simulink model "usrp_fm_fdm"  (R2014b)
settings: Solver=ode45  StartTime=0.0  StopTime=inf  RelTol=1e-3
PreLoadFcn:
  | %%%%%%%%%%%%%%%%%%%%%%%%%%%%%%%%%%%%%%%%%%%%%%%%%%%%%%%%%%%%%%%%%%%%%%%%%%%
  | % check to see if Simulink library folder is missing from the MATLAB path %
  | %%%%%%%%%%%%%%%%%%%%%%%%%%%%%%%%%%%%%%%%%%%%%%%%%%%%%%%%%%%%%%%%%%%%%%%%%%%
  | if isempty(strfind(path, 'rtlsdr_book_library'))
  | 
  |     % create error window
  |     fig_error = figure(...
  |         'Name', 'Error: RTL-SDR Book Library',...
  |         'Toolbar','none',...
  |         'MenuBar','none',...
  |         'NumberTitle','off',...
  |         'Resize','off',...
  |         'WindowStyle','modal');
  |     fig_error.Position(3) = 600;
  |     fig_error.Position(4) = 150;
  |     fig_axes = axes(...
  |         'Parent',fig_error,...
  |         'Position',[0,0,1,1],...
  |         'visible','off');
  |     % error message
  |     t_title = text(.05,.8,...
  |         'MISSING DIRECTORIES',...
  |         'FontSize',11.5);
  |     t_body = text(.075,.6,...
  |         [{'Simulink cannot find the  \it{<root>}\rm / \it{rtlsdr\_book\_library}\rm  folder in the \it{MATLAB Path}\rm.'},...
  |         {'Please set the MATLAB path following the instructions given in Exercise 2.4.'}],...
  |         'FontSize',10.5);
  |     % buttons
  |     btn_path = uicontrol(...
  |         'Parent',fig_error,...
  |         'String','Set Path Now',...
  |         'FontSize',10,...
  |         'Callback', 'pathtool; close(fig_error);',...
  |         'Position', [fig_error.Position(3)/2-210, 30, 200, 30]);
  |     btn_abort = uicontrol(...
  |         'Parent',fig_error,...
  |         'String','No thanks',...
  |         'FontSize',10,...
  |         'Callback', 'close(fig_error); abort=1;',...
  |         'Position', [fig_error.Position(3)/2+10, 30, 200, 30]);
  | 
  |     % pause to allow user to interact with error box
  |     uiwait(fig_error);
  | 
  |     % abort simulation
  |     try
  |         if abort==1
  |             set_param(gcs, 'SimulationCommand', 'stop');
  |         end
  |     end
  | 
  |     % if user has set path, allow diagram to be updated
  |     if ~exist('abort','var')
  |         % create error window
  |         fig_update = figure(...
  |             'Name', 'Update Diagram',...
  |             'Toolbar','none',...
  |             'MenuBar','none',...
  |             'NumberTitle','off',...
  |             'Resize','off');
  |         fig_update.Position(3) = 400;
  |         fig_update.Position(4) = 120;
  |         fig_axes = axes(...
  |             'Parent',fig_update,...
  |             'Position',[0,0,1,1],...
  |             'visible','off');
  |         % instruction message
  |         t_body = text(.075,.7,...
  |             'Once you have set the path, update the block diagram',...
  |             'FontSize',10.5);
  |         % button
  |         btn_update = uicontrol(...
  |             'Parent',fig_update,...
  |             'String','Update Block Diagram',...
  |             'FontSize',10,...
  |             'Callback', 'set_param(gcs,''SimulationCommand'',''update''); close(gcf)',...
  |             'Position', [fig_update.Position(3)/2-100, 30, 200, 30]);
  |     end
  | 
  |     % clear error components
  |     clear('fig_error','fig_update','fig_axes','t_title','t_body','btn_path','btn_abort','btn_update','abort');
  | 
  | end
  | %%%%%%%%%%%%%%%%%%%%%%%%%%%%%%%%%%%%%%%%%%%%%%%%%%%%%%%%%%%%%%%%%%%%%%%%%%%
undefined symbols (not defined in the file): dfilt, fdesignblkfcn, gcbh, startfcn_spectrum_analyzer
libraries: dsparch4 x9, dspmlti4 x4, dspvision x4, dspsrcs4 x4, dspmtrx3 x2, rtlsdr_book_library x1, commsdrhw_v2 x1
(part 1 of 2)
CloseFcn:
  | closefcn_model
Description:
  | Software, Simulation Examples and Design Exercises Licence Agreement
  | 
  | This license agreement refers to the simulation examples, design exercises and files,
  | and associated software MATLAB and Simulink resources that accompany the book:
  | 
  |      Title: Software Defined Radio using MATLAB & Simulink and the RTL-SDR
  |      Published by Strathclyde Academic Media, 2015
  |      Authored by Robert W. Stewart, Kenneth W. Barlee, Dale S.W. Atkinson,
  |      and Louise H. Crockett
  | 
  | and made available as a download from, www.desktopSDR.com or variously acquired
  | by other means such as via USB storage, cloud storage, disk or any other electronic
  | or optical or magnetic storage mechanism. These files and associated software may
  | be used subject to the terms of agreement of the conditions below:
  | 
  |     Copyright © 2015 Robert W. Stewart, Kenneth W. Barlee, Dale S.W. Atkinson,
  |     and Louise H. Crockett
  |     All rights reserved.
  | 
  | Redistribution and use in source and binary forms, with or without modification, are
  | permitted provided that the following conditions are met:
  | 
  |    1.  Redistributions of source code must retain the above copyright notice, this list of
  |         conditions and the following disclaimer.
  | 
  |    2.  Redistributions in binary form must reproduce the above copyright notice, this
  |         list of conditions and the following disclaimer in the documentation and/or other
  |         materials provided with the distribution.
  | 
  |    3.  Neither the name of the copyright holder nor the names of its contributors may
  |         be used to endorse or promote products derived from this software without
  |         specific prior written permission.
  | 
  |    4.  In all cases, the software is, and all modifications and derivatives of the
  |         software shall be, licensed to you solely for use in conjunction with The
  |         MathWorks, Inc. products and service offerings.
  | 
  | THIS SOFTWARE IS PROVIDED BY THE COPYRIGHT HOLDERS AND CONTRIBUTORS
  | "AS IS" AND ANY EXPRESS OR IMPLIED WARRANTIES, INCLUDING, BUT NOT LIMITED
  | TO, THE IMPLIED WARRANTIES OF MERCHANTABILITY AND FITNESS FOR A
  | PARTICULAR PURPOSE ARE DISCLAIMED. IN NO EVENT SHALL THE COPYRIGHT
  | HOLDER OR CONTRIBUTORS BE LIABLE FOR ANY DIRECT, INDIRECT, INCIDENTAL,
  | SPECIAL, EXEMPLARY, OR CONSEQUENTIAL DAMAGES (INCLUDING, BUT NOT
  | LIMITED TO, PROCUREMENT OF SUBSTITUTE GOODS OR SERVICES; LOSS OF USE,
  | DATA, OR PROFITS; OR BUSINESS INTERRUPTION) HOWEVER CAUSED AND ON ANY
  | THEORY OF LIABILITY, WHETHER IN CONTRACT, STRICT LIABILITY, OR TORT
  | (INCLUDING NEGLIGENCE OR OTHERWISE) ARISING IN ANY WAY OUT OF THE USE
  | OF THIS SOFTWARE, EVEN IF ADVISED OF THE POSSIBILITY OF SUCH DAMAGE.
  | 
  | 
  | Audio Tracks used in Simulations Examples and Design Exercises
  | 
  | The music and vocal files used within the Examples files and software within the book
  | were variously written, arranged, performed, recorded and produced by Garrey Rice,
  | Adam Struth, Jamie Struth, Iain Thistlethwaite and also Marshall Craigmyle who
  | collectively, and individually where appropriate, assert and retain all of their copyright,
  | performance and artistic rights. Permission to use and reproduce this music is
  | granted for all purposes associated with MATLAB and Simulink software and the
  | simulation examples and design exercises files that accompany this book. Requests to
  | use the music for any other purpose should be directed to: info@desktopSDR.com.
  | For information on music track names, full credits, and links to the musicians please
  | refer to www.desktopSDR.com/more/audio.
settings Model: SimulationMode=accelerator  Creator=desktopSDR Team  LastModifiedBy=desktopSDR Team
settings DataIOCC: LimitDataPoints=off  SaveOutput=off  SignalLogging=off  SaveTime=off

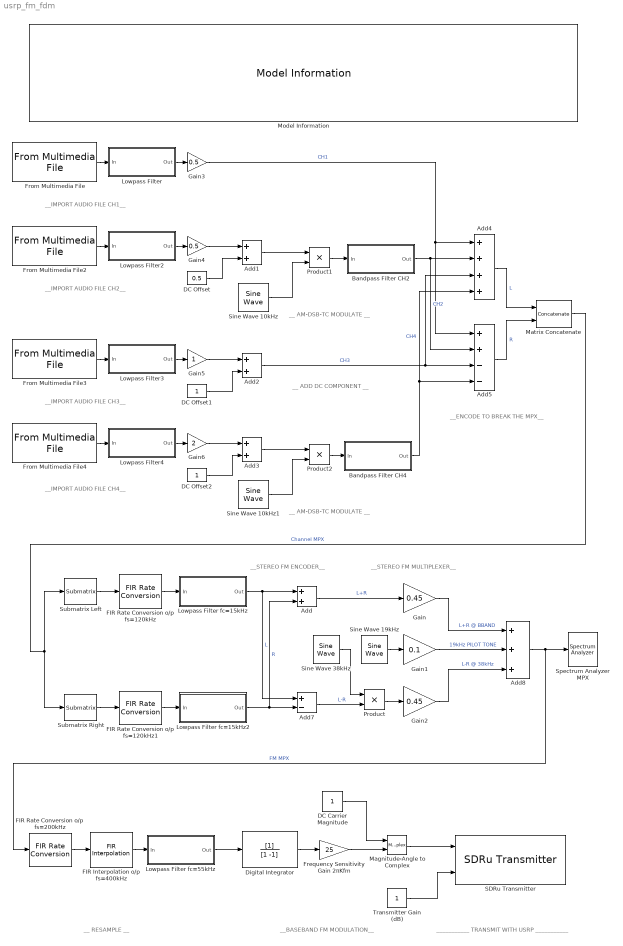
== system usrp_fm_fdm ==
  note: __ AM-DSB-TC MODULATE __
  note: __ AM-DSB-TC MODULATE __
  note: __ ADD DC COMPONENT __
  note: __IMPORT AUDIO FILE CH1__
  note: __IMPORT AUDIO FILE CH2__
  note: __IMPORT AUDIO FILE CH3__
  note: __IMPORT AUDIO FILE CH4__
  note: __ENCODE TO BREAK THE MPX__
  note: __STEREO FM MULTIPLEXER__
  note: __STEREO FM ENCODER__
  note: __ RESAMPLE __
  note: ___________ TRANSMIT WITH USRP ___________
  note: __BASEBAND FM MODULATION__
  Add{,1..3} (4 alike) : Sum
  Add4 : Sum  Inputs=++++
  Add5 : Sum  Inputs=++--
  Add7 : Sum  Inputs=+-
  Add8 : Sum  Inputs=+++
  Bandpass Filter CH2 : Subsystem  DialogController=fdesignblkfcn  InitFcn=fdesignblkfcn(gcbh, {'InitFcn'});  mask(Bandpass Filter){}
      mask help: Design a bandpass filter
      settings: CopyFcn=fdesignblkfcn(gcbh, {'CopyFcn'});
      mask Help: helpview(mapfilelocation('dsp'), 'dspbandpassfilter');
      mask Display: disp('Bandpass');
  Bandpass Filter CH4 : Subsystem  DialogController=fdesignblkfcn  InitFcn=fdesignblkfcn(gcbh, {'InitFcn'});  mask(Bandpass Filter){}
      mask help: Design a bandpass filter
      settings: CopyFcn=fdesignblkfcn(gcbh, {'CopyFcn'});
      mask Help: helpview(mapfilelocation('dsp'), 'dspbandpassfilter');
      mask Display: disp('Bandpass');
  DC Carrier Magnitude : Constant
  DC Offset : Constant  Value=0.5
  DC Offset1 : Constant
  DC Offset2 : Constant
  Digital Integrator : DiscreteFilter  Denominator=[1 -1]  InputProcessing=Columns as channels (frame based)  FilterStructure=Direct form II transposed  a0EqualsOne=on
  FIR Interpolation o/p fs=400kHz : dspmlti4/FIR Interpolation  h=firpm(100, [0 53e3 65e3 400e3/2]/(400e3/2), [1 1 0 0], [1 1],20)  L=2  framing=Allow multirate processing  outputBufInitCond=0  InputProcessing=Columns as channels (frame based)  firstCoeffDataTypeStr=Inherit: Same word length as input  firstCoeffLastDataTypeStr=Inherit: Same word length as input  firstCoeffMin=[]  firstCoeffMax=[]  outputDataTypeStr=Inherit: Same as accumulator  outputLastDataTypeStr=Inherit: Same as accumulator  outputMin=[]  outputMax=[]  roundingMode=Floor  overflowMode=off  FilterSource=Specify via dialog  FilterObject=Hm_firinterp
  FIR Rate Conversion o/p fs=120kHz : dspmlti4/FIR Rate Conversion  L=5  h=firpm(250, [0 15e3 20e3 240e3/2]/(240e3/2), [1 1 0 0], [1 1],20)  M=2  firstCoeffDataTypeStr=Inherit: Same word length as input  firstCoeffLastDataTypeStr=Inherit: Same word length as input  firstCoeffMin=[]  firstCoeffMax=[]  outputDataTypeStr=Inherit: Same as accumulator  outputLastDataTypeStr=Inherit: Same as accumulator  outputMin=[]  outputMax=[]  roundingMode=Floor  overflowMode=off  FilterSource=Specify via dialog  FilterObject=Hm_firsrc
  FIR Rate Conversion o/p fs=120kHz1 : dspmlti4/FIR Rate Conversion  L=5  h=firpm(250, [0 15e3 20e3 240e3/2]/(240e3/2), [1 1 0 0], [1 1],20)  M=2  firstCoeffDataTypeStr=Inherit: Same word length as input  firstCoeffLastDataTypeStr=Inherit: Same word length as input  firstCoeffMin=[]  firstCoeffMax=[]  outputDataTypeStr=Inherit: Same as accumulator  outputLastDataTypeStr=Inherit: Same as accumulator  outputMin=[]  outputMax=[]  roundingMode=Floor  overflowMode=off  FilterSource=Specify via dialog  FilterObject=Hm_firsrc
  FIR Rate Conversion o/p fs=200kHz : dspmlti4/FIR Rate Conversion  L=5  h=firpm(200, [0 53e3 65e3 600e3/2]/(600e3/2), [1 1 0 0], [1 1],20)  M=3  firstCoeffDataTypeStr=Inherit: Same word length as input  firstCoeffLastDataTypeStr=Inherit: Same word length as input  firstCoeffMin=[]  firstCoeffMax=[]  outputDataTypeStr=Inherit: Same as accumulator  outputLastDataTypeStr=Inherit: Same as accumulator  outputMin=[]  outputMax=[]  roundingMode=Floor  overflowMode=off  FilterSource=Specify via dialog  FilterObject=Hm_firsrc
  Frequency Sensitivity Gain 2πKfm : Gain  Gain=25
  From Multimedia File : dspvision/From Multimedia File  inputFilename=../../audio_sources/music1_mono48kHz.wav  loop=on  numPlays=inf  outputStreams=Audio only  videoDataType=single  audioDataType=double  inheritSampleTime=on  userDefinedSampleTime=1/30  noAudioOutput=off  isIntensityVideo=off  fourcc=RGB  colorVideoFormat=Separate color signals  outputEOF=off  dataOrg=Column-major  audioFrameSize=600  computeAudioFrameSize=off  outSamplingMode=Frame based
  From Multimedia File2 : dspvision/From Multimedia File  inputFilename=../../audio_sources/music2_mono48kHz.wav  loop=on  numPlays=inf  outputStreams=Audio only  videoDataType=single  audioDataType=double  inheritSampleTime=on  userDefinedSampleTime=1/30  noAudioOutput=off  isIntensityVideo=off  fourcc=RGB  colorVideoFormat=Separate color signals  outputEOF=off  dataOrg=Column-major  audioFrameSize=600  computeAudioFrameSize=off  outSamplingMode=Frame based
  From Multimedia File3 : dspvision/From Multimedia File  inputFilename=../../audio_sources/music3_mono48kHz.wav  loop=on  numPlays=inf  outputStreams=Audio only  videoDataType=single  audioDataType=double  inheritSampleTime=on  userDefinedSampleTime=1/30  noAudioOutput=off  isIntensityVideo=off  fourcc=RGB  colorVideoFormat=Separate color signals  outputEOF=off  dataOrg=Column-major  audioFrameSize=600  computeAudioFrameSize=off  outSamplingMode=Frame based
  From Multimedia File4 : dspvision/From Multimedia File  inputFilename=../../audio_sources/music4_mono48kHz.wav  loop=on  numPlays=inf  outputStreams=Audio only  videoDataType=single  audioDataType=double  inheritSampleTime=on  userDefinedSampleTime=1/30  noAudioOutput=off  isIntensityVideo=off  fourcc=RGB  colorVideoFormat=Separate color signals  outputEOF=off  dataOrg=Column-major  audioFrameSize=600  computeAudioFrameSize=off  outSamplingMode=Frame based
  Gain : Gain  Gain=0.45
  Gain1 : Gain  Gain=0.1
  Gain2 : Gain  Gain=0.45
  Gain3 : Gain  Gain=0.5
  Gain4 : Gain  Gain=0.5
  Gain5 : Gain
  Gain6 : Gain  Gain=2
  Lowpass Filter : Subsystem  DialogController=fdesignblkfcn  InitFcn=fdesignblkfcn(gcbh, {'InitFcn'});  mask(Lowpass Filter){}
      mask help: Design a lowpass filter
      settings: CopyFcn=fdesignblkfcn(gcbh, {'CopyFcn'});
      mask Help: helpview(mapfilelocation('dsp'), 'dsplowpassfilter');
      mask Display: disp('Lowpass')
  Lowpass Filter fc=15kHz : Subsystem  DialogController=fdesignblkfcn  InitFcn=fdesignblkfcn(gcbh, {'InitFcn'});  mask(Lowpass Filter){}
      mask help: Design a lowpass filter
      settings: CopyFcn=fdesignblkfcn(gcbh, {'CopyFcn'});
      mask Help: helpview(mapfilelocation('dsp'), 'dsplowpassfilter');
      mask Display: disp('Lowpass')
  Lowpass Filter fc=15kHz2 : Subsystem  DialogController=fdesignblkfcn  InitFcn=fdesignblkfcn(gcbh, {'InitFcn'});  mask(Lowpass Filter){}
      mask help: Design a lowpass filter
      settings: CopyFcn=fdesignblkfcn(gcbh, {'CopyFcn'});
      mask Help: helpview(mapfilelocation('dsp'), 'dsplowpassfilter');
      mask Display: disp('Lowpass')
  Lowpass Filter fc=55kHz : Subsystem  DialogController=fdesignblkfcn  InitFcn=fdesignblkfcn(gcbh, {'InitFcn'});  mask(Lowpass Filter){}
      mask help: Design a lowpass filter
      settings: CopyFcn=fdesignblkfcn(gcbh, {'CopyFcn'});
      mask Help: helpview(mapfilelocation('dsp'), 'dsplowpassfilter');
      mask Display: disp('Lowpass')
  Lowpass Filter2 : Subsystem  DialogController=fdesignblkfcn  InitFcn=fdesignblkfcn(gcbh, {'InitFcn'});  mask(Lowpass Filter){}
      mask help: Design a lowpass filter
      settings: CopyFcn=fdesignblkfcn(gcbh, {'CopyFcn'});
      mask Help: helpview(mapfilelocation('dsp'), 'dsplowpassfilter');
      mask Display: disp('Lowpass')
  Lowpass Filter3 : Subsystem  DialogController=fdesignblkfcn  InitFcn=fdesignblkfcn(gcbh, {'InitFcn'});  mask(Lowpass Filter){}
      mask help: Design a lowpass filter
      settings: CopyFcn=fdesignblkfcn(gcbh, {'CopyFcn'});
      mask Help: helpview(mapfilelocation('dsp'), 'dsplowpassfilter');
      mask Display: disp('Lowpass')
  Lowpass Filter4 : Subsystem  DialogController=fdesignblkfcn  InitFcn=fdesignblkfcn(gcbh, {'InitFcn'});  mask(Lowpass Filter){}
      mask help: Design a lowpass filter
      settings: CopyFcn=fdesignblkfcn(gcbh, {'CopyFcn'});
      mask Help: helpview(mapfilelocation('dsp'), 'dsplowpassfilter');
      mask Display: disp('Lowpass')
  Magnitude-Angle to Complex : MagnitudeAngleToComplex
  Matrix Concatenate : Concatenate  Mode=Multidimensional array  ConcatenateDimension=2
  Model Information : rtlsdr_book_library/Additional Tools/Model Information/Model Information
  Product : Product
  Product1 : Product
  Product2 : Product
  SDRu Transmitter : commsdrhw_v2/SDRu Transmitter  rxtx=tx  platform=N200/N210/USRP2  USRP2_IP='169.254.10.2'  USRP_IP_X300='192.168.10.2'  USRP_IP_X310='192.168.10.2'  USRP_serialNumB200=''  USRP_serialNumB210=''  centerFrequency=433.9e6  centerFrequencySrc=Dialog  loOffset=1.5e6  loOffsetSrc=Dialog  masterClkRateB200=32e6  masterClkRateB210=32e6  masterClkRateX300=200e6  masterClkRateX310=200e6  masterClkRateParam=100e6  gain=10  gainSrc=Input port  decimInterp=250  decimInterpSrc=Dialog  USRP2_IP_NUM=[49 54 57 46 50 53 52 46 49 48 46 50]  frameLength=362  outputDatatype=int16  overrunUnderrunPort=off  sampleTime=1  dboardInfo=|  HOST_DATA_PORT=30000  HOST_CONTROL_PORT=30001  USRP2_DATA_PORT=32769  USRP2_CONTROL_PORT=32768  bufferMode=Continuous streaming  EnableBurstMode=off  NumFramesInBurst=100  USRP_ID='169.254.10.2'
      | dbid: 0
      |           dbName: 'no db found'
      |          freqMin: 0
      |          freqMax: 0
      |          gainMin: 0
      |          gainMax: 0
      |     gainStepSize: 0
  Sine Wave 10kHz : dspsrcs4/Sine Wave  Amplitude=1  Frequency=10e3  Phase=0  SampleMode=Discrete  OutComplex=Real  CompMethod=Trigonometric fcn  TableSize=Speed  SampleTime=1/48e3  SamplesPerFrame=600  ResetState=Restart at time zero  dataType=double  wordLen=16  udDataType=sfix(16)  fracBitsMode=Best precision  numFracBits=15  OutDataTypeStr=double  LastOutDataTypeStr=double
  Sine Wave 10kHz1 : dspsrcs4/Sine Wave  Amplitude=1  Frequency=10e3  Phase=0  SampleMode=Discrete  OutComplex=Real  CompMethod=Trigonometric fcn  TableSize=Speed  SampleTime=1/48e3  SamplesPerFrame=600  ResetState=Restart at time zero  dataType=double  wordLen=16  udDataType=sfix(16)  fracBitsMode=Best precision  numFracBits=15  OutDataTypeStr=double  LastOutDataTypeStr=double
  Sine Wave 19kHz : dspsrcs4/Sine Wave  Amplitude=1  Frequency=19e3  Phase=0  SampleMode=Discrete  OutComplex=Real  CompMethod=Trigonometric fcn  TableSize=Speed  SampleTime=1/120e3  SamplesPerFrame=1500  ResetState=Restart at time zero  dataType=double  wordLen=16  udDataType=sfix(16)  fracBitsMode=Best precision  numFracBits=15  OutDataTypeStr=double  LastOutDataTypeStr=double
  Sine Wave 38kHz : dspsrcs4/Sine Wave  Amplitude=1  Frequency=38e3  Phase=0  SampleMode=Discrete  OutComplex=Real  CompMethod=Trigonometric fcn  TableSize=Speed  SampleTime=1/120e3  SamplesPerFrame=1500  ResetState=Restart at time zero  dataType=double  wordLen=16  udDataType=sfix(16)  fracBitsMode=Best precision  numFracBits=15  OutDataTypeStr=double  LastOutDataTypeStr=double
  Spectrum Analyzer MPX : SpectrumAnalyzer  StartFcn=startfcn_spectrum_analyzer;
  Submatrix Left : dspmtrx3/Submatrix  RowSpan=All rows  RowStartMode=First  RowStartIndex=1  RowEndMode=Last  RowEndIndex=1  ColSpan=One column  ColStartMode=First  ColStartIndex=1  ColEndMode=Last  ColEndIndex=1
  Submatrix Right : dspmtrx3/Submatrix  RowSpan=All rows  RowStartMode=First  RowStartIndex=1  RowEndMode=Last  RowEndIndex=1  ColSpan=One column  ColStartMode=Last  ColStartIndex=1  ColEndMode=Last  ColEndIndex=1
  Transmitter Gain (dB) : Constant
  wires:
  From Multimedia File/1 -> Lowpass Filter/1(In)
  From Multimedia File2/1 -> Lowpass Filter2/1(In)
  Gain3/1 -> Add5/1, Add4/1  "CH1"
  Matrix Concatenate/1 -> Submatrix Right/1, Submatrix Left/1  "Channel MPX"
  Bandpass Filter CH2/1(Out) -> Add5/2, Add4/2  "CH2"
  Sine Wave 10kHz/1 -> Product1/2
  Lowpass Filter2/1(Out) -> Gain4/1
  Lowpass Filter/1(Out) -> Gain3/1
  Add4/1 -> Matrix Concatenate/1  "L"
  From Multimedia File3/1 -> Lowpass Filter3/1(In)
  From Multimedia File4/1 -> Lowpass Filter4/1(In)
  Add2/1 -> Add4/3, Add5/3  "CH3"
  Bandpass Filter CH4/1(Out) -> Add4/4, Add5/4  "CH4"
  Add5/1 -> Matrix Concatenate/2  "R"
  Digital Integrator/1 -> Frequency Sensitivity Gain 2πKfm/1
  DC Carrier Magnitude/1 -> Magnitude-Angle to Complex/1
  Frequency Sensitivity Gain 2πKfm/1 -> Magnitude-Angle to Complex/2
  FIR Rate Conversion o/p fs=200kHz/1 -> FIR Interpolation o/p fs=400kHz/1
  Submatrix Left/1 -> FIR Rate Conversion o/p fs=120kHz/1
  Magnitude-Angle to Complex/1 -> SDRu Transmitter/1
  Transmitter Gain (dB)/1 -> SDRu Transmitter/2
  FIR Interpolation o/p fs=400kHz/1 -> Lowpass Filter fc=55kHz/1(In)
  FIR Rate Conversion o/p fs=120kHz/1 -> Lowpass Filter fc=15kHz/1(In)
  FIR Rate Conversion o/p fs=120kHz1/1 -> Lowpass Filter fc=15kHz2/1(In)
  Add/1 -> Gain/1  "L+R"
  Add7/1 -> Product/2  "L-R"
  Gain/1 -> Add8/1  "L+R @ BBAND"
  Lowpass Filter fc=15kHz2/1(Out) -> Add/2, Add7/2  "R"
  Lowpass Filter fc=15kHz/1(Out) -> Add/1, Add7/1  "L"
  Sine Wave 38kHz/1 -> Product/1
  Product/1 -> Gain2/1
  Sine Wave 19kHz/1 -> Gain1/1
  Gain1/1 -> Add8/2  "19kHz PILOT TONE"
  Gain2/1 -> Add8/3  "L-R @ 38kHz"
  Add8/1 -> Spectrum Analyzer MPX/1, FIR Rate Conversion o/p fs=200kHz/1  "FM MPX"
  Lowpass Filter fc=55kHz/1(Out) -> Digital Integrator/1
  Product1/1 -> Bandpass Filter CH2/1(In)
  DC Offset/1 -> Add1/2
  Gain4/1 -> Add1/1
  Add1/1 -> Product1/1
  Lowpass Filter3/1(Out) -> Gain5/1
  Sine Wave 10kHz1/1 -> Product2/2
  Lowpass Filter4/1(Out) -> Gain6/1
  Product2/1 -> Bandpass Filter CH4/1(In)
  DC Offset2/1 -> Add3/2
  Gain6/1 -> Add3/1
  Add3/1 -> Product2/1
  DC Offset1/1 -> Add2/2
  Gain5/1 -> Add2/1
  Submatrix Right/1 -> FIR Rate Conversion o/p fs=120kHz1/1

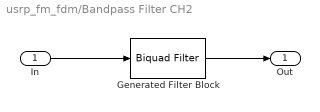
== system usrp_fm_fdm/Bandpass Filter CH2 ==
  In : Inport
  Generated Filter Block : dsparch4/Biquad Filter  Tag=BlockMethodSubSystem  IIRFiltStruct=Direct form II  CoeffSource=Specify via dialog  BiQuadCoeffs=[0.038316192503797628 0 -0.038316192503797628 1 -1.4647964271306382 0.94471193100608086;0.079066094669843018 0 -0.079066094669843018 1 -1.4478872277903871 0.92340777287438502;1.4987829140143916 0 -1.4987829140143916 1 -1.3806603018180277 0.84224281947976043;1.4262911444791151 0 -1.4262911444791151 1 0.58822635838518289 0.83492615482033594;0.12651868683152687 0 -0.12651868683152687 1 0.55132638249904864 0.75583004259253694;0.16278534730934821 0 -0.16278534730934821 1 -1.2966897472444947 0.74843901978838634;0.17165110687366142 0 -0.17165110687366142 1 -1.2286258519522211 0.67826050546120453;1.2698273089041128 0 -1.2698273089041128 1 -1.2113783161788541 0.66128071032184788;0.20679428223229873 0 -0.20679428223229873 1 0.45755483002581882 0.59529881813215735;0.24203724548995573 0 -0.24203724548995573 1 -1.1410250658492758 0.59529322698110076;0.25085765032621543 0 -0.25085765032621543 1 -1.0676878443588242 0.53197037847147466;1.126279711749548 0 -1.126279711749548 1 -1.0487453100276105 0.51650173917589026;0.28689353541085899 0 -0.28689353541085899 1 0.35194175339474887 0.46218165129526712;0.32503837865501967 0 -0.32503837865501967 1 -0.96986311471358477 0.45593385510682533;1.0469924746795094 0 -1.0469924746795094 1 -0.88468241094327671 0.39740220475460497;0.36600529716476377 0 -0.36600529716476377 1 0.28503939659387545 0.39655389906045352;0.97025355161809246 0 -0.97025355161809246 1 -0.79108046931960774 0.34121276752547225;0.41170205075459598 0 -0.41170205075459598 1 0.21209573444104943 0.33805385051512005;0.89433754435568558 0 -0.89433754435568558 1 -0.68658006847610853 0.28850567166718427;0.81944502214294834 0 -0.81944502214294834 1 0.13161626710115268 0.28686560436176478;0.46356432779720524 0 -0.46356432779720524 1 0.04162240295248873 0.24384468958098351;0.74310982737617426 0 -0.74310982737617426 1 -0.56911862362598731 0.24200449865234019;0.52401642408429905 0 -0.52401642408429905 1 -0.060257140448974872 0.21085064512665347;0.66634747068770672 0 -0.66634747068770672 1 -0.43950658142365717 0.20676604963866144;0.59171836614561379 0 -0.59171836614561379 1 -0.17601055769180649 0.19112080655833777;0.62712191993186395 0 -0.62712191993186395 1 -0.30478008617749786 0.1889115855767009;0.6996674218388591 0 -0.6996674218388591 1 -0.23904135382384295 0.18757452699095289;0.5533055925452488 0 -0.5533055925452488 1 -0.11634228576068448 0.19906897851393116;0.7691707424752533 0 -0.7691707424752533 1 -0.37209094308052626 0.19536146214396241;0.4861749900243762 0 -0.4861749900243762 1 -0.0076804609149881825 0.22592720694312432;0.83504112081969384 0 -0.83504112081969384 1 -0.50556036680048488 0.22257689527031296;0.42757746379429407 0 -0.42757746379429407 1 0.087951306871739909 0.26424643599944614;0.37860716298259472 0 -0.37860716298259472 1 -0.62953035756411846 0.26422094963295606;0.85794319827651022 0 -0.85794319827651022 1 -0.74034910133001608 0.31430206283391698;0.31567823731936401 0 -0.31567823731936401 1 0.17290986841503597 0.31151116853219291;0.72504748895787763 0 -0.72504748895787763 1 -0.83908419359333841 0.36896989749244552;0.68432655624176875 0 -0.68432655624176875 1 0.24940543484309963 0.36641429161510974;0.31152694401360886 0 -0.31152694401360886 1 0.31916944212687015 0.42846811137787677;0.68648839199988665 0 -0.68648839199988665 1 -0.92818196779966999 0.42640778321597261;0.30752809817970561 0 -0.30752809817970561 1 0.38347969139959959 0.49774535746443022;0.27169501816632519 0 -0.27169501816632519 1 -1.0099766818316462 0.48596263367743714;0.77277817453089559 0 -0.77277817453089559 1 -1.1048021701758266 0.56332975000387675;0.73508031520028017 0 -0.73508031520028017 1 0.4286923007015444 0.55473049811770825;0.29418562251053348 0 -0.29418562251053348 1 0.48546564941124559 0.63808189197476139;0.23621087503198029 0 -0.23621087503198029 1 -1.1765054758560756 0.62792026806225021;0.92057985047504287 0 -0.92057985047504287 1 -1.26281575076854 0.71287380301019321;0.19821400336650971 0 -0.19821400336650971 1 0.52563846635605771 0.70676158328244509 ...(+4904 chars)Flag=Warning  IC=0  ICnum=0  ICden=0  InputProcessing=Columns as channels (frame based)  denAccumFracLength=30  denProdOutputFracLength=30  secondMemoryFracLength=15  roundingMode=Floor  overflowMode=off  ScaleValues=[0.036348121033666261;1;1;1;1;1;1;1;1;1;1;1;1;1;1;1;1;1;1;1;1;1;1;1;1;1;1;1;1;1;1;1;1;1;1;1;1;1;1;1;1;1;1;1;1;1;1;1;1;1;1;1;1;1;1;1;1;1;1;1;1;1;1;1;1;1;1;1;1;1;1;1;1;1;1;1;1;1;1;1;1;1;1;1;1;1;1;1;1;1;1;1;1;1;1;1;1;1;1;1;1;1;1;1;1;1]  optimizeScaleValues=off  ScaleValueMode=Specify via input port (g)  scaleValueFracLength=14  FilterSource=Specify via dialog  dfiltObjectName=dfilt.df2tsos([1 0.3 0.4],[1 0.1 0.2])
  Out : Outport
  wires:
  In/1 -> Generated Filter Block/1
  Generated Filter Block/1 -> Out/1

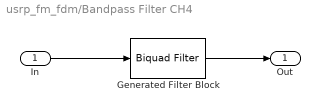
== system usrp_fm_fdm/Bandpass Filter CH4 ==
  In : Inport
  Generated Filter Block : dsparch4/Biquad Filter  Tag=BlockMethodSubSystem  IIRFiltStruct=Direct form II  CoeffSource=Specify via dialog  BiQuadCoeffs=[0.038316192503797628 0 -0.038316192503797628 1 -1.4647964271306382 0.94471193100608086;0.079066094669843018 0 -0.079066094669843018 1 -1.4478872277903871 0.92340777287438502;1.4987829140143916 0 -1.4987829140143916 1 -1.3806603018180277 0.84224281947976043;1.4262911444791151 0 -1.4262911444791151 1 0.58822635838518289 0.83492615482033594;0.12651868683152687 0 -0.12651868683152687 1 0.55132638249904864 0.75583004259253694;0.16278534730934821 0 -0.16278534730934821 1 -1.2966897472444947 0.74843901978838634;0.17165110687366142 0 -0.17165110687366142 1 -1.2286258519522211 0.67826050546120453;1.2698273089041128 0 -1.2698273089041128 1 -1.2113783161788541 0.66128071032184788;0.20679428223229873 0 -0.20679428223229873 1 0.45755483002581882 0.59529881813215735;0.24203724548995573 0 -0.24203724548995573 1 -1.1410250658492758 0.59529322698110076;0.25085765032621543 0 -0.25085765032621543 1 -1.0676878443588242 0.53197037847147466;1.126279711749548 0 -1.126279711749548 1 -1.0487453100276105 0.51650173917589026;0.28689353541085899 0 -0.28689353541085899 1 0.35194175339474887 0.46218165129526712;0.32503837865501967 0 -0.32503837865501967 1 -0.96986311471358477 0.45593385510682533;1.0469924746795094 0 -1.0469924746795094 1 -0.88468241094327671 0.39740220475460497;0.36600529716476377 0 -0.36600529716476377 1 0.28503939659387545 0.39655389906045352;0.97025355161809246 0 -0.97025355161809246 1 -0.79108046931960774 0.34121276752547225;0.41170205075459598 0 -0.41170205075459598 1 0.21209573444104943 0.33805385051512005;0.89433754435568558 0 -0.89433754435568558 1 -0.68658006847610853 0.28850567166718427;0.81944502214294834 0 -0.81944502214294834 1 0.13161626710115268 0.28686560436176478;0.46356432779720524 0 -0.46356432779720524 1 0.04162240295248873 0.24384468958098351;0.74310982737617426 0 -0.74310982737617426 1 -0.56911862362598731 0.24200449865234019;0.52401642408429905 0 -0.52401642408429905 1 -0.060257140448974872 0.21085064512665347;0.66634747068770672 0 -0.66634747068770672 1 -0.43950658142365717 0.20676604963866144;0.59171836614561379 0 -0.59171836614561379 1 -0.17601055769180649 0.19112080655833777;0.62712191993186395 0 -0.62712191993186395 1 -0.30478008617749786 0.1889115855767009;0.6996674218388591 0 -0.6996674218388591 1 -0.23904135382384295 0.18757452699095289;0.5533055925452488 0 -0.5533055925452488 1 -0.11634228576068448 0.19906897851393116;0.7691707424752533 0 -0.7691707424752533 1 -0.37209094308052626 0.19536146214396241;0.4861749900243762 0 -0.4861749900243762 1 -0.0076804609149881825 0.22592720694312432;0.83504112081969384 0 -0.83504112081969384 1 -0.50556036680048488 0.22257689527031296;0.42757746379429407 0 -0.42757746379429407 1 0.087951306871739909 0.26424643599944614;0.37860716298259472 0 -0.37860716298259472 1 -0.62953035756411846 0.26422094963295606;0.85794319827651022 0 -0.85794319827651022 1 -0.74034910133001608 0.31430206283391698;0.31567823731936401 0 -0.31567823731936401 1 0.17290986841503597 0.31151116853219291;0.72504748895787763 0 -0.72504748895787763 1 -0.83908419359333841 0.36896989749244552;0.68432655624176875 0 -0.68432655624176875 1 0.24940543484309963 0.36641429161510974;0.31152694401360886 0 -0.31152694401360886 1 0.31916944212687015 0.42846811137787677;0.68648839199988665 0 -0.68648839199988665 1 -0.92818196779966999 0.42640778321597261;0.30752809817970561 0 -0.30752809817970561 1 0.38347969139959959 0.49774535746443022;0.27169501816632519 0 -0.27169501816632519 1 -1.0099766818316462 0.48596263367743714;0.77277817453089559 0 -0.77277817453089559 1 -1.1048021701758266 0.56332975000387675;0.73508031520028017 0 -0.73508031520028017 1 0.4286923007015444 0.55473049811770825;0.29418562251053348 0 -0.29418562251053348 1 0.48546564941124559 0.63808189197476139;0.23621087503198029 0 -0.23621087503198029 1 -1.1765054758560756 0.62792026806225021;0.92057985047504287 0 -0.92057985047504287 1 -1.26281575076854 0.71287380301019321;0.19821400336650971 0 -0.19821400336650971 1 0.52563846635605771 0.70676158328244509 ...(+4904 chars)Flag=Warning  IC=0  ICnum=0  ICden=0  InputProcessing=Columns as channels (frame based)  denAccumFracLength=30  denProdOutputFracLength=30  secondMemoryFracLength=15  roundingMode=Floor  overflowMode=off  ScaleValues=[0.036348121033666261;1;1;1;1;1;1;1;1;1;1;1;1;1;1;1;1;1;1;1;1;1;1;1;1;1;1;1;1;1;1;1;1;1;1;1;1;1;1;1;1;1;1;1;1;1;1;1;1;1;1;1;1;1;1;1;1;1;1;1;1;1;1;1;1;1;1;1;1;1;1;1;1;1;1;1;1;1;1;1;1;1;1;1;1;1;1;1;1;1;1;1;1;1;1;1;1;1;1;1;1;1;1;1;1;1]  optimizeScaleValues=off  ScaleValueMode=Specify via input port (g)  scaleValueFracLength=14  FilterSource=Specify via dialog  dfiltObjectName=dfilt.df2tsos([1 0.3 0.4],[1 0.1 0.2])
  Out : Outport
  wires:
  In/1 -> Generated Filter Block/1
  Generated Filter Block/1 -> Out/1

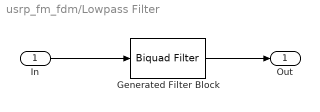
== system usrp_fm_fdm/Lowpass Filter ==
  In : Inport
  Generated Filter Block : dsparch4/Biquad Filter  Tag=BlockMethodSubSystem  IIRFiltStruct=Direct form II  CoeffSource=Specify via dialog  BiQuadCoeffs=[0.02505658453151734 0.050113169063034681 0.02505658453151734 1 -1.6618358052504689 0.92327518660477159;0.037716014607021689 0.075432029214043378 0.037716014607021689 1 -1.5666197180702381 0.81307974054400167;0.048494542600695072 0.096989085201390143 0.048494542600695072 1 -1.483833787366122 0.71726995848240305;0.057562689362794101 0.1151253787255882 0.057562689362794101 1 -1.4124095756411101 0.63460931673938947;0.065066669960849324 0.13013333992169865 0.065066669960849324 1 -1.3513355886493104 0.5639271931762575;0.071126049882347511 0.14225209976469502 0.071126049882347511 1 -1.2996951874675289 0.50416274358054824;0.075826965263644491 0.15165393052728898 0.075826965263644491 1 -1.2566848480829704 0.45438603384519421;0.079207708097762716 0.15841541619552543 0.079207708097762716 1 -1.2216205877683222 0.41380547733850032;0.081213644661423695 0.16242728932284739 0.081213644661423695 1 -1.1939377721788489 0.38176761165383055;0.08148106483340975 0.1629621296668195 0.08148106483340975 1 -1.1731876770814522 0.35775311943117882;0.076637308661870573 0.15327461732374115 0.076637308661870573 1 -1.1590329311748637 0.34137155424355531;0.047546496662289287 0.095092993324578573 0.047546496662289287 1 -1.1512431451247189 0.3323562819935113;0.04540058431321875 0.090801168626437501 0.04540058431321875 1 -1.1496915016555413 0.3305605345596806;0.045831247000341468 0.091662494000682937 0.045831247000341468 1 -1.1543527405881076 0.3359550778409825;0.046516257123944797 0.093032514247889594 0.046516257123944797 1 -1.1653027462029997 0.34862773420436555;0.047466760014933662 0.094933520029867324 0.047466760014933662 1 -1.1827197756415799 0.36878480413735909;0.048698191344618065 0.09739638268923613 0.048698191344618065 1 -1.2068872094697505 0.39675424952948513;0.050230457593599342 0.10046091518719868 0.050230457593599342 1 -1.2381975142107695 0.43299027958924174;0.052088101393404251 0.1041762027868085 0.052088101393404251 1 -1.2771568309371673 0.47807866131156473;0.054300385989436643 0.10860077197887329 0.054300385989436643 1 -1.3243891792379572 0.53274158481157419;0.056901193140924844 0.11380238628184969 0.056901193140924844 1 -1.3806386047689676 0.59784014872671409;0.059928568932260555 0.11985713786452111 0.059928568932260555 1 -1.4467665832625731 0.6743713558262725;0.063423665332839996 0.12684733066567999 0.063423665332839996 1 -1.5237404723519465 0.76345474808098879;0.023993836801624483 0.047987673603248966 0.023993836801624483 1 -1.612606599730263 0.86630126106162297;0.014199710532717848 0.028399421065435696 0.014199710532717848 1 -1.7144385404499303 0.98415336424243371;0.028453803345255303 0.056907606690510606 0.028453803345255303 1 -1.6368075882726612 0.89430953998294882;0.04083171761385794 0.08166343522771588 0.04083171761385794 1 -1.5448001049050344 0.78782747407497666;0.051459392354549008 0.10291878470909802 0.051459392354549008 1 -1.4649534370622368 0.69541935859814075;0.060531990296125222 0.12106398059225044 0.060531990296125222 1 -1.3962083671487442 0.61585934024476119;0.06815377125244737 0.13630754250489474 0.06815377125244737 1 -1.3375744913620335 0.54800120526008977;0.074455848419753085 0.14891169683950617 0.074455848419753085 1 -1.2881623105057174 0.49081551877004753;0.079552479596548167 0.15910495919309633 0.079552479596548167 1 -1.2471979145071224 0.44340661946156557;0.083510197687583193 0.16702039537516639 0.083510197687583193 1 -1.2140273488611264 0.40501767295371627;0.086395360489223874 0.17279072097844775 0.086395360489223874 1 -1.1881153515668013 0.37502921002970635;0.08825814050628647 0.17651628101257294 0.08825814050628647 1 -1.1690414739763555 0.35295463721924042;0.072653340568011524 0.14530668113602305 0.072653340568011524 1 -1.1564954726095342 0.33843490365490059;0.10631278825624907 0.21262557651249814 0.10631278825624907 1 -1.150273121708774 0.33123365486006179;0.09066349956390464 0.09066349956390464 0 1 -0.57474884697500372 0;0.045700079748393248 0.091400159496786496 0.045700079748393248 1 -1.1526025576110279 ...(+1167 chars)Flag=Warning  IC=0  ICnum=0  ICden=0  InputProcessing=Columns as channels (frame based)  denAccumFracLength=30  denProdOutputFracLength=30  secondMemoryFracLength=15  roundingMode=Floor  overflowMode=off  ScaleValues=[0.038531123333914737;1;1;1;1;1;1;1;1;1;1;1;1;1;1;1;1;1;1;1;1;1;1;1;1;1;1;1;1;1;1;1;1;1;1;1;1;1;1;1;1;1;1;1;1;1;1;1;1;1;1]  optimizeScaleValues=off  ScaleValueMode=Specify via input port (g)  scaleValueFracLength=14  FilterSource=Specify via dialog  dfiltObjectName=dfilt.df2tsos([1 0.3 0.4],[1 0.1 0.2])
  Out : Outport
  wires:
  In/1 -> Generated Filter Block/1
  Generated Filter Block/1 -> Out/1

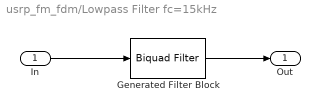
== system usrp_fm_fdm/Lowpass Filter fc=15kHz ==
  In : Inport
  Generated Filter Block : dsparch4/Biquad Filter  Tag=BlockMethodSubSystem  IIRFiltStruct=Direct form II  CoeffSource=Specify via dialog  BiQuadCoeffs=[0.47317005345169666 -0.30307728548160168 0.3552862054548247 1 -1.3238737006712475 0.86511185339799446;0.25407991836614779 0.013136135916053305 0.00082836158684250797 1 -1.5734734560410242 0.70525008464109618;0.26098132032063748 -0.29548649035134594 0.034572981551380208 1 -1.3156763282103388 0.66891715813083463;0.030797704742965809 -0.0062470044848620589 0.0024961066929451189 1 -1.3942015618174157 0.77798854949818474;1.5211188179161075 -2 1.5075788908074403 1 -1.3865253012495609 0.98071245573948018;-0.86987276178120643 0.55655777437114651 -0.25149509973734757 1 -1.357338185996994 0.84525618519026846;0.25557566805887638 0.14108303077480563 0.19172424260597029 1 -1.6306553480127399 0.68783931627099504;0.1592819381000054 0.076004983723057917 0.0061187770260567554 1 -1.8253479266443986 0.82545247207677486;0.07934261365834086 -0.0022173795904536437 0.045369159306579282 1 -1.4840124255643086 0.72683648922007227;1.6187100875684302 -2 1.5743866150788544 1 -1.3664078844337517 0.93151058917172236]  a0Flag=Warning  IC=0  ICnum=0  ICden=0  InputProcessing=Columns as channels (frame based)  denAccumFracLength=30  denProdOutputFracLength=30  secondMemoryFracLength=15  roundingMode=Floor  overflowMode=off  ScaleValues=[0.094760439304554744;1;1;1;1;1;1;1;1;1;3.8950302415849745]  optimizeScaleValues=off  ScaleValueMode=Specify via input port (g)  scaleValueFracLength=14  FilterSource=Specify via dialog  dfiltObjectName=dfilt.df2tsos([1 0.3 0.4],[1 0.1 0.2])
  Out : Outport
  wires:
  In/1 -> Generated Filter Block/1
  Generated Filter Block/1 -> Out/1
